simulink model "LevelandTemperature"  (R2013a)
settings: Solver=ode45  StartTime=0.0  StopTime=10.0  RelTol=1e-3
settings Model: Creator=haresh  LastModifiedBy=haresh

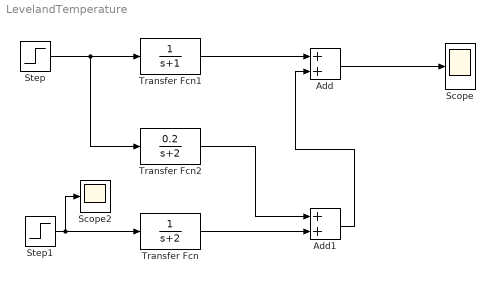
== system LevelandTemperature ==
  Add : Sum
  Add1 : Sum
  Scope : Scope
      settings: TimeRange=100
  Scope2 : Scope
      settings: SaveName=ScopeData2
  Step : Step  Time=0  SampleTime=0
  Step1 : Step  Time=10  SampleTime=0
  Transfer Fcn : TransferFcn  Denominator=[1 2]
  Transfer Fcn1 : TransferFcn  Denominator=[1 1]
  Transfer Fcn2 : TransferFcn  Numerator=[0.2]  Denominator=[1 2]
  wires:
  Step/1 -> Transfer Fcn2/1, Transfer Fcn1/1
  Step1/1 -> Transfer Fcn/1, Scope2/1
  Transfer Fcn/1 -> Add1/2
  Transfer Fcn2/1 -> Add1/1
  Transfer Fcn1/1 -> Add/1
  Add1/1 -> Add/2
  Add/1 -> Scope/1
